simulink model "sl_subsys_fcncall7"  (Simulink 7.6)
settings: Solver=FixedStepDiscrete  StartTime=0.0  StopTime=10.0  FixedStep=0.1  RelTol=1e-3
Description:
  | Enabled subsystem containing function-call subsystems that specify state and output reset behavior
  | 
  | The enabled subsystem below contains two function-call subsystems.
  | The left function-call subsystem is configured to hold the value
  | of its states upon enable, and to hold the value of its output upon
  | disable.  The right function-call subsystem is configured to reset
  | the value of its states upon enable, and to reset the value of its
  | output upon disable.
settings Model: Creator=The MathWorks Inc.  CovMetricSettings=d  ExtModeAutoUpdateStatusClock=off
settings DataIOCC: SignalLoggingName=logsOut
settings OptimizationCC: BlockReduction=off  BooleanDataType=off  InlineInvariantSignals=on  InitFltsAndDblsToZero=on
settings DebuggingCC: SaveWithParameterizedLinksMsg=none  CheckExecutionContextPreStartOutputMsg=on  CheckExecutionContextRuntimeOutputMsg=on  SignalResolutionControl=TryResolveAllWithWarning  SolverPrmCheckMsg=none  MultiTaskDSMMsg=warning  MultiTaskCondExecSysMsg=none
settings HardwareCC: TargetUnknown=on
settings ModelReferenceCC: UpdateModelReferenceTargets=IfOutOfDate
settings SFSimCC: SimParseCustomCode=off
settings RTWCC: IncludeERTFirstTime=on
settings CodeAppCC: CustomSymbolStrFcn=$F$N$M
settings GRTTargetCC: TargetFcnLib=ansi_tfl_tmw.mat

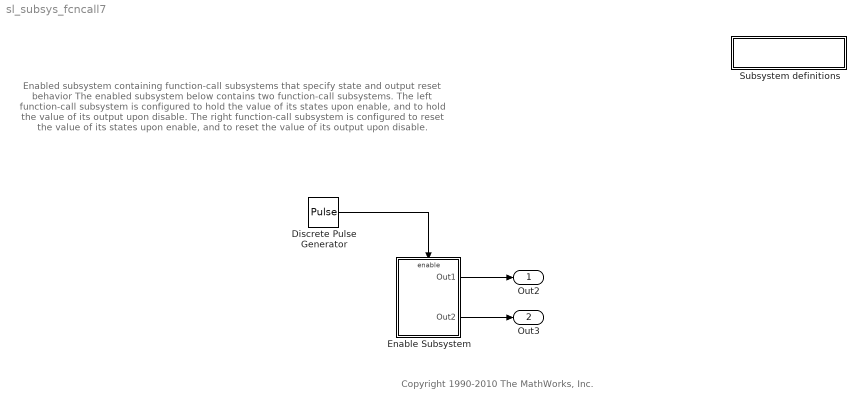
== system sl_subsys_fcncall7 ==
  note: Enabled subsystem containing function-call subsystems that specify
      | state and output reset behavior
      |
      | The enabled subsystem below contains two function-call subsystems.
      | The left function-call subsystem is configured to hold the value
      | of its states upon enable, and to hold the value of its output upon
      | disable.  The right function-call subsystem is configured to reset
      | the value of its states upon enable, and to reset the value of its
      | output upon disable.
  note: Copyright 1990-2010 The MathWorks, Inc.
  " Subsystem definitions" : Subsystem
      settings: OpenFcn=helpview([matlabroot,'/toolbox/simulink/simdemos/simfeatures/html/sl_subsys_definitions.html']);
      mask Display: disp('Subsystem\ndefinitions')
  Discrete Pulse Generator : DiscretePulseGenerator  Period=20  PulseWidth=10  SampleTime=0.1
  Enable Subsystem : Subsystem  TreatAsAtomicUnit=on
  Out2 : Outport
  Out3 : Outport  Port=2
  wires:
  Enable Subsystem/1(Out1) -> Out2/1
  Discrete Pulse Generator/1 -> Enable Subsystem/Enable
  Enable Subsystem/2(Out2) -> Out3/1

== system sl_subsys_fcncall7/ Subsystem definitions ==

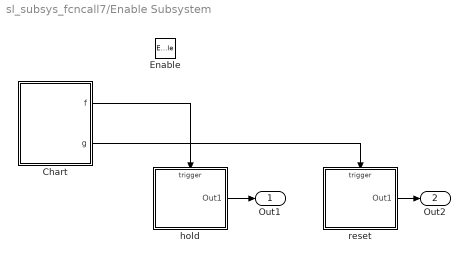
== system sl_subsys_fcncall7/Enable Subsystem ==
  Enable : EnablePort
  Chart : Stateflow chart  TreatAsAtomicUnit=on
  hold : Subsystem  TreatAsAtomicUnit=on
  reset : Subsystem  TreatAsAtomicUnit=on
  Out1 : Outport
  Out2 : Outport  Port=2
  wires:
  Chart/1(f) -> hold/Trigger
  Chart/2(g) -> reset/Trigger
  hold/1(Out1) -> Out1/1
  reset/1(Out1) -> Out2/1

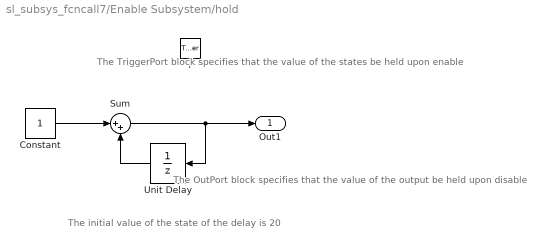
== system sl_subsys_fcncall7/Enable Subsystem/hold ==
  note: The initial value of the state of the delay is 20
  note: The OutPort block
      | specifies that the value
      | of the output be held
      | upon disable
  note: The TriggerPort block
      | specifies that the value
      | of the states be held
      | upon enable
  f : TriggerPort  TriggerType=function-call
  Constant : Constant
  Sum : Sum  Inputs=|++  SaturateOnIntegerOverflow=on  InputSameDT=on  OutDataTypeStr=Inherit: Same as first input
  Unit Delay : UnitDelay  X0=20  SampleTime=-1
  Out1 : Outport
  wires:
  Sum/1 -> Unit Delay/1, Out1/1
  Unit Delay/1 -> Sum/2
  Constant/1 -> Sum/1

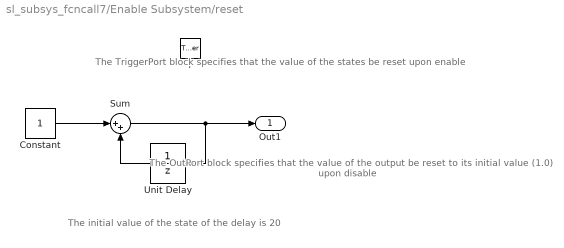
== system sl_subsys_fcncall7/Enable Subsystem/reset ==
  note: The TriggerPort block
      | specifies that the value
      | of the states be reset
      | upon enable
  note: The OutPort block
      | specifies that the value
      | of the output be reset
      | to its initial value (1.0)
      | upon disable
  note: The initial value of the state of the delay is 20
  f : TriggerPort  TriggerType=function-call  StatesWhenEnabling=reset
  Constant : Constant
  Sum : Sum  Inputs=|++  SaturateOnIntegerOverflow=on  InputSameDT=on  OutDataTypeStr=Inherit: Same as first input
  Unit Delay : UnitDelay  X0=20  SampleTime=-1
  Out1 : Outport  OutputWhenDisabled=reset  InitialOutput=1
  wires:
  Constant/1 -> Sum/1
  Unit Delay/1 -> Sum/2
  Sum/1 -> Out1/1, Unit Delay/1

== stateflow chart Enable Subsystem/Chart ==
  settings: updateMethod=DISCRETE  sampleTime=0.1
  state one/
    entry: f;
  state two/
    entry: g;
  one -> two
  two -> one
  (default) -> one
  events: f output FUNCTION_CALL_EVENT; g output FUNCTION_CALL_EVENT
